simulink model "ex_2"  (R2023a)
settings: Solver=FixedStepAuto  StartTime=0.0  StopTime=1  FixedStep=1e-4  RelTol=1e-3
libraries: simulink x1
settings Model: Creator=LabCom  LastModifiedBy=LabCom

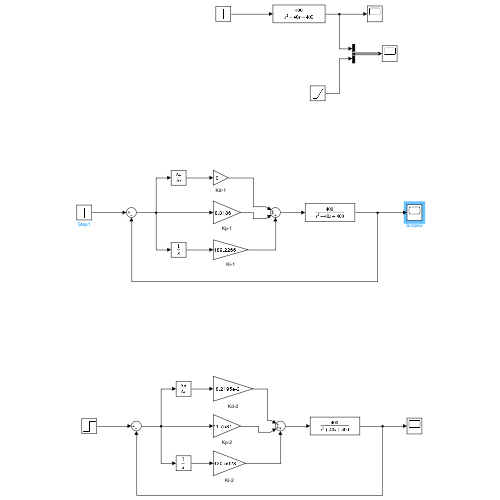
[thumbnail: Simulink's stored preview of the top-level diagram]
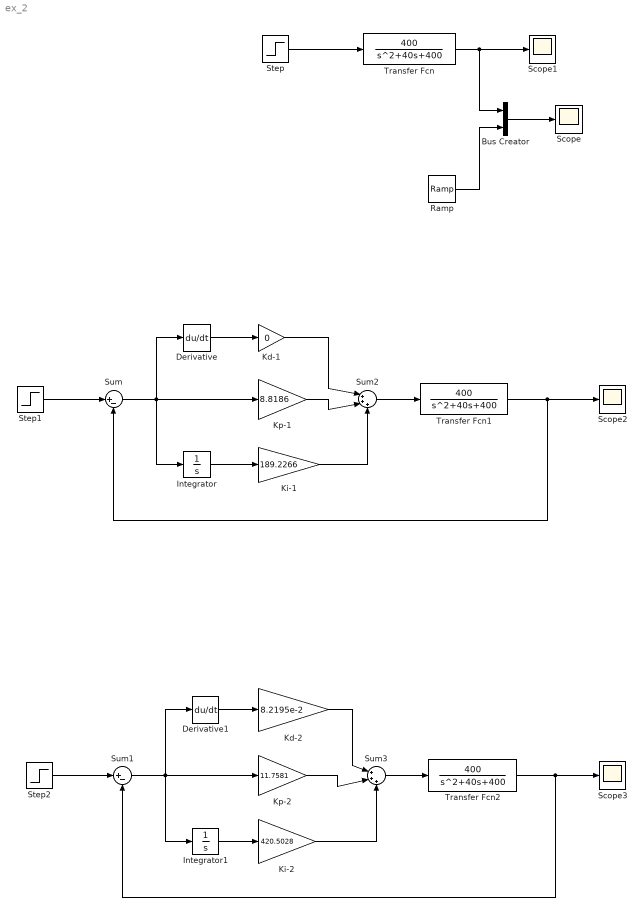
== system ex_2 ==
  Bus Creator : BusCreator  Inputs=2
  Derivative : Derivative
  Derivative1 : Derivative
  Integrator : Integrator
  Integrator1 : Integrator
  Kd-1 : Gain  Gain=0
  Kd-2 : Gain  Gain=8.2195e-2
  Ki-1 : Gain  Gain=189.2266
  Ki-2 : Gain  Gain=420.5028
  Kp-1 : Gain  Gain=8.8186
  Kp-2 : Gain  Gain=11.7581
  Ramp : simulink/Sources/Ramp  slope=7.2997  start=1.3981e-2  InitialOutput=0
  Scope{,1..3} (4 alike) : Scope
  Step : Step  Time=0  SampleTime=0
  Step1 : Step  Time=0  SampleTime=0
  Step2 : Step  Time=0  SampleTime=0
  Sum : Sum  Inputs=|+-
  Sum1 : Sum  Inputs=|+-
  Sum2 : Sum  Inputs=|+++
  Sum3 : Sum  Inputs=|+++
  Transfer Fcn : TransferFcn  Numerator=[400]  Denominator=[1 40 400]
  Transfer Fcn1 : TransferFcn  Numerator=[400]  Denominator=[1 40 400]
  Transfer Fcn2 : TransferFcn  Numerator=[400]  Denominator=[1 40 400]
  wires:
  Step/1 -> Transfer Fcn/1
  Transfer Fcn/1 -> Scope1/1, Bus Creator/1
  Bus Creator/1 -> Scope/1
  Ramp/1 -> Bus Creator/2
  Derivative/1 -> Kd-1/1
  Kd-1/1 -> Sum2/1
  Ki-1/1 -> Sum2/3
  Integrator/1 -> Ki-1/1
  Step1/1 -> Sum/1
  Sum2/1 -> Transfer Fcn1/1
  Sum/1 -> Derivative/1, Kp-1/1, Integrator/1
  Transfer Fcn1/1 -> Scope2/1, Sum/2
  Kp-1/1 -> Sum2/2
  Sum1/1 -> Derivative1/1, Kp-2/1, Integrator1/1
  Step2/1 -> Sum1/1
  Kp-2/1 -> Sum3/2
  Transfer Fcn2/1 -> Scope3/1, Sum1/2
  Ki-2/1 -> Sum3/3
  Integrator1/1 -> Ki-2/1
  Derivative1/1 -> Kd-2/1
  Kd-2/1 -> Sum3/1
  Sum3/1 -> Transfer Fcn2/1
